simulink library "Surface_Profile_Axle3_zx"  (R2025b)
settings: Solver=VariableStepAuto  StartTime=0.0  StopTime=10.0  RelTol=1e-3
Description:
  | Simscape Vehicle Templates Library
  | 
  | Copyright 2018-2025 The MathWorks, Inc.
settings Model: Creator=smiller  LastModifiedBy=smiller
settings ModelReferenceCC: EnableRefExpFcnMdlSchedulingChecks=on
settings RTWCC: GPUComputeCapability=3.5

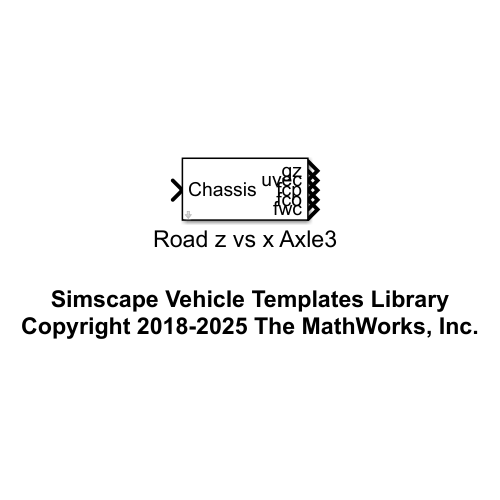
[thumbnail: Simulink's stored preview of the top-level diagram]
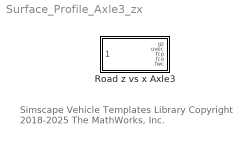
== system Surface_Profile_Axle3_zx ==
  note: Simscape Vehicle Templates Library
      | Copyright 2018-2025 The MathWorks, Inc.
  Road z vs x Axle3 : Subsystem  VariantControl=Variant  mask{dist_x=flipud(Scene.RDF_Plateau.Road.extr_data_L(45:end,1)), height_z=flipud(Scene.RDF_Plateau.Road.extr_data_L(45:end,2))}
      mask prompts: dist_x "Distance vector [x] (m)"; height_z "Height vector [z] (m)"
      mask init:
      | pitch_rd = atan2(circshift(height_z,-2)-circshift(height_z,2),circshift(dist_x,-2)-circshift(dist_x,2));
      | pitch_rd(1:2) = pitch_rd(3);
      | pitch_rd(end-1:end) = pitch_rd(end-2);

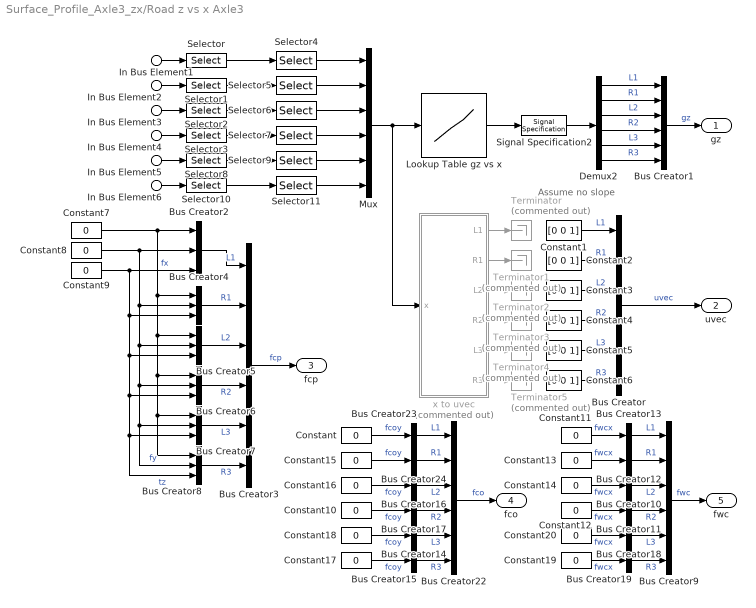
== system Surface_Profile_Axle3_zx/Road z vs x Axle3 ==
  note: Assume no slope
  In Bus Element1 : Inport  PortName=Chassis  Element=WhlL1.xyz
  In Bus Element2 : Inport  PortName=Chassis  Element=WhlR1.xyz
  In Bus Element3 : Inport  PortName=Chassis  Element=WhlL2.xyz
  In Bus Element4 : Inport  PortName=Chassis  Element=WhlR2.xyz
  In Bus Element5 : Inport  PortName=Chassis  Element=WhlL3.xyz
  In Bus Element6 : Inport  PortName=Chassis  Element=WhlR3.xyz
  Bus Creator{,1,3,9,22} (5 alike) : BusCreator  Inputs=6
  Bus Creator{10..19,23..24} (12 alike) : BusCreator  Inputs=1
  Bus Creator{2,4..8} (6 alike) : BusCreator  Inputs=3
  Constant{,7..20} (15 alike) : Constant  Value=0
  Constant{1..6} (6 alike) : Constant  Value=[0 0 1]
  Demux2 : Demux  Outputs=6
  Lookup Table gz vs x : Lookup_n-D  NumberOfTableDimensions=1  BreakpointsForDimension1=dist_x  Table=height_z  InternalRulePriority=Speed  RndMeth=Simplest
  Mux : Mux  Inputs=6
  Selector{,1..3,8,10} (6 alike) : Selector  InputPortWidth=3  IndexOptions=Index vector (dialog)  Indices=[1 2]  OutputSizes=1
  Selector{4..7,9,11} (6 alike) : Selector  InputPortWidth=2  IndexOptions=Index vector (dialog)  Indices=1  OutputSizes=1
  Signal Specification2 : SignalSpecification  Unit=m
  Terminator{,1..5} (6 alike) : Terminator  Commented=on
  x to uvec : Subsystem  Commented=on
  gz : Outport  VectorParamsAs1DForOutWhenUnconnected=off
  uvec : Outport  Port=2  VectorParamsAs1DForOutWhenUnconnected=off
  fcp : Outport  Port=3  VectorParamsAs1DForOutWhenUnconnected=off
  fco : Outport  Port=4  VectorParamsAs1DForOutWhenUnconnected=off
  fwc : Outport  Port=5  VectorParamsAs1DForOutWhenUnconnected=off
  wires:
  x to uvec/6(R3) -> Terminator5/1
  x to uvec/5(L3) -> Terminator4/1
  Demux2/6 -> Bus Creator1/6  "R3"
  Demux2/5 -> Bus Creator1/5  "L3"
  Constant6/1 -> Bus Creator/6  "R3"
  Constant5/1 -> Bus Creator/5  "L3"
  Selector10/1 -> Selector11/1
  In Bus Element6/1 -> Selector10/1
  Selector11/1 -> Mux/6
  Selector9/1 -> Mux/5
  In Bus Element5/1 -> Selector8/1
  Selector8/1 -> Selector9/1
  Lookup Table gz vs x/1 -> Signal Specification2/1
  Mux/1 -> x to uvec/1(x), Lookup Table gz vs x/1
  Selector4/1 -> Mux/1
  Selector5/1 -> Mux/2
  Selector6/1 -> Mux/3
  Selector7/1 -> Mux/4
  Selector3/1 -> Selector7/1
  Selector2/1 -> Selector6/1
  Selector1/1 -> Selector5/1
  Selector/1 -> Selector4/1
  In Bus Element4/1 -> Selector3/1
  In Bus Element2/1 -> Selector1/1
  In Bus Element1/1 -> Selector/1
  In Bus Element3/1 -> Selector2/1
  Demux2/3 -> Bus Creator1/3  "L2"
  Signal Specification2/1 -> Demux2/1
  Demux2/2 -> Bus Creator1/2  "R1"
  Demux2/1 -> Bus Creator1/1  "L1"
  Demux2/4 -> Bus Creator1/4  "R2"
  Bus Creator1/1 -> gz/1  "gz"
  Bus Creator/1 -> uvec/1  "uvec"
  Constant1/1 -> Bus Creator/1  "L1"
  x to uvec/1(L1) -> Terminator/1
  x to uvec/2(R1) -> Terminator1/1
  x to uvec/3(L2) -> Terminator2/1
  x to uvec/4(R2) -> Terminator3/1
  Constant2/1 -> Bus Creator/2  "R1"
  Constant3/1 -> Bus Creator/3  "L2"
  Constant4/1 -> Bus Creator/4  "R2"
  Bus Creator7/1 -> Bus Creator3/5  "L3"
  Constant8/1 -> Bus Creator2/2, Bus Creator4/2, Bus Creator5/2, Bus Creator6/2, Bus Creator7/2, Bus Creator8/2  "fy"
  Constant7/1 -> Bus Creator2/1, Bus Creator4/1, Bus Creator5/1, Bus Creator8/1, Bus Creator7/1, Bus Creator6/1  "fx"
  Bus Creator8/1 -> Bus Creator3/6  "R3"
  Bus Creator4/1 -> Bus Creator3/2  "R1"
  Bus Creator2/1 -> Bus Creator3/1  "L1"
  Bus Creator6/1 -> Bus Creator3/4  "R2"
  Bus Creator5/1 -> Bus Creator3/3  "L2"
  Bus Creator3/1 -> fcp/1  "fcp"
  Constant9/1 -> Bus Creator2/3, Bus Creator4/3, Bus Creator5/3, Bus Creator6/3, Bus Creator7/3, Bus Creator8/3  "tz"
  Constant20/1 -> Bus Creator18/1  "fwcx"
  Constant13/1 -> Bus Creator12/1  "fwcx"
  Constant15/1 -> Bus Creator24/1  "fcoy"
  Bus Creator10/1 -> Bus Creator9/3  "L2"
  Constant10/1 -> Bus Creator17/1  "fcoy"
  Bus Creator13/1 -> Bus Creator9/1  "L1"
  Bus Creator23/1 -> Bus Creator22/1  "L1"
  Bus Creator17/1 -> Bus Creator22/4  "R2"
  Constant14/1 -> Bus Creator10/1  "fwcx"
  Bus Creator22/1 -> fco/1  "fco"
  Constant17/1 -> Bus Creator15/1  "fcoy"
  Bus Creator15/1 -> Bus Creator22/6  "R3"
  Bus Creator14/1 -> Bus Creator22/5  "L3"
  Bus Creator18/1 -> Bus Creator9/5  "L3"
  Constant12/1 -> Bus Creator11/1  "fwcx"
  Bus Creator9/1 -> fwc/1  "fwc"
  Constant18/1 -> Bus Creator14/1  "fcoy"
  Bus Creator19/1 -> Bus Creator9/6  "R3"
  Bus Creator24/1 -> Bus Creator22/2  "R1"
  Constant16/1 -> Bus Creator16/1  "fcoy"
  Bus Creator16/1 -> Bus Creator22/3  "L2"
  Constant19/1 -> Bus Creator19/1  "fwcx"
  Constant11/1 -> Bus Creator13/1  "fwcx"
  Constant/1 -> Bus Creator23/1  "fcoy"
  Bus Creator12/1 -> Bus Creator9/2  "R1"
  Bus Creator11/1 -> Bus Creator9/4  "R2"

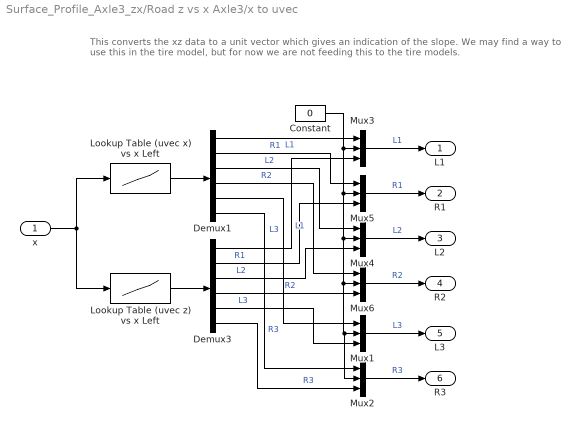
== system Surface_Profile_Axle3_zx/Road z vs x Axle3/x to uvec ==
  note: This converts the xz data to a unit vector which gives an indication of the slope. We may find a way to use this in the tire model, but for now we are not feeding this to the tire models.
  x : Inport
  Constant : Constant  Value=0
  Demux1 : Demux  Outputs=6
  Demux3 : Demux  Outputs=6
  Lookup Table (uvec x) vs x Left : Lookup_n-D  NumberOfTableDimensions=1  BreakpointsForDimension1=dist_x  Table=sin(pitch_rd)  InternalRulePriority=Speed  RndMeth=Simplest
  Lookup Table (uvec z) vs x Left : Lookup_n-D  NumberOfTableDimensions=1  BreakpointsForDimension1=dist_x  Table=cos(pitch_rd)  InternalRulePriority=Speed  RndMeth=Simplest
  Mux{1..6} (6 alike) : Mux  Inputs=3
  L1 : Outport  VectorParamsAs1DForOutWhenUnconnected=off
  R1 : Outport  Port=2  VectorParamsAs1DForOutWhenUnconnected=off
  L2 : Outport  Port=3  VectorParamsAs1DForOutWhenUnconnected=off
  R2 : Outport  Port=4  VectorParamsAs1DForOutWhenUnconnected=off
  L3 : Outport  Port=5  VectorParamsAs1DForOutWhenUnconnected=off
  R3 : Outport  Port=6  VectorParamsAs1DForOutWhenUnconnected=off
  wires:
  Demux3/6 -> Mux2/3  "R3"
  Demux3/5 -> Mux1/3  "L3"
  Demux1/6 -> Mux2/1  "R3"
  Demux1/5 -> Mux1/1  "L3"
  Mux1/1 -> L3/1  "L3"
  Mux2/1 -> R3/1  "R3"
  x/1 -> Lookup Table (uvec x) vs x Left/1, Lookup Table (uvec z) vs x Left/1
  Mux6/1 -> R2/1  "R2"
  Demux1/2 -> Mux5/1  "R1"
  Demux1/3 -> Mux4/1  "L2"
  Lookup Table (uvec z) vs x Left/1 -> Demux3/1
  Mux3/1 -> L1/1  "L1"
  Constant/1 -> Mux6/2, Mux1/2, Mux2/2, Mux4/2, Mux5/2, Mux3/2
  Lookup Table (uvec x) vs x Left/1 -> Demux1/1
  Demux3/3 -> Mux4/3  "L2"
  Mux5/1 -> R1/1  "R1"
  Demux1/1 -> Mux3/1  "L1"
  Demux3/2 -> Mux5/3  "R1"
  Demux3/4 -> Mux6/3  "R2"
  Demux1/4 -> Mux6/1  "R2"
  Demux3/1 -> Mux3/3  "L1"
  Mux4/1 -> L2/1  "L2"
